simulink model "pattern_separation"  (R2019b)
settings: Solver=FixedStepAuto  StartTime=1  StopTime=simulationtime  FixedStep=stepsize  RelTol=1e-3
values from neighbouring files (symbols this model uses):
  a1 = 0.02    [simulation.m]
  a2 = 0.02    [simulation.m]
  b1 = 0.025    [simulation.m]
  b2 = 0.04    [simulation.m]
  c1 = -65    [simulation.m]
  C1 = normrnd(100,10,[1,nrofgranulecells])    [simulation.m]
  c2 = -65    [simulation.m]
  C2 = normrnd(100,10,[1,nrofinterneurons])    [simulation.m]
  d1 = 6    [simulation.m]
  d2 = 2    [simulation.m]
  inputset = inputsets{no_input}    [simulation.m]
  k1 = 0.25    [simulation.m]
  k2 = 0.25    [simulation.m]
  minimum_saturation_limit_1 = -80    [simulation.m]
  minimum_saturation_limit_2 = -100    [simulation.m]
  noumberofevents = 500    [simulation.m]
  Re = 230    [simulation.m]
  simulationtime = 2000    [simulation.m]
  stepsize = 1    [simulation.m]
  ve1 = -5    [simulation.m]
  ve2 = -80    [simulation.m]
  vr1 = -60    [simulation.m]
  vr2 = -65    [simulation.m]
  vt1 = -55    [simulation.m]
  vt2 = -48    [simulation.m]
undefined symbols (not defined in the file or in its folder): conductancemaxima1, conductancemaxima2, conductancemaxima3, decaytimes1, decaytimes2, decaytimes3, DiscIntNeverNeededParam, Nd, trace
(part 2 of 5)

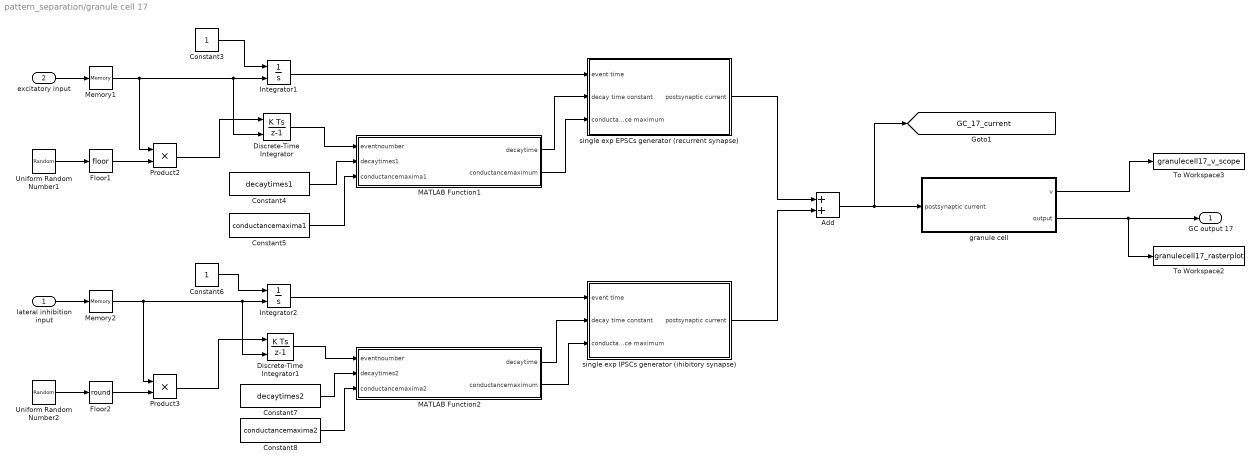
== system pattern_separation/granule cell 17 ==
  lateral inhibition input : Inport
  excitatory input : Inport  Port=2
  Add : Sum
  Constant3 : Constant  SampleTime=-1
  Constant4 : Constant  Value=decaytimes1  SampleTime=-1
  Constant5 : Constant  Value=conductancemaxima1  SampleTime=-1
  Constant6 : Constant  SampleTime=-1
  Constant7 : Constant  Value=decaytimes2  SampleTime=-1
  Constant8 : Constant  Value=conductancemaxima2  SampleTime=-1
  Discrete-Time Integrator : DiscreteIntegrator  gainval=1/stepsize  ExternalReset=sampled level  SampleTime=-1  ICPrevOutput=DiscIntNeverNeededParam  ICPrevScaledInput=DiscIntNeverNeededParam
  Discrete-Time Integrator1 : DiscreteIntegrator  gainval=1/stepsize  ExternalReset=sampled level  SampleTime=-1  ICPrevOutput=DiscIntNeverNeededParam  ICPrevScaledInput=DiscIntNeverNeededParam
  Floor1 : Rounding
  Floor2 : Rounding  Operator=round
  Integrator1 : Integrator  ExternalReset=level hold
  Integrator2 : Integrator  ExternalReset=level hold
  MATLAB Function1 : MATLAB Function  TreatAsAtomicUnit=on
  MATLAB Function2 : MATLAB Function  TreatAsAtomicUnit=on
  Memory1 : Memory  InheritSampleTime=on
  Memory2 : Memory  InheritSampleTime=on
  Product2 : Product
  Product3 : Product
  To Workspace2 : ToWorkspace  VariableName=granulecell17_rasterplot  SampleTime=-1
  To Workspace3 : ToWorkspace  VariableName=granulecell17_v_scope  SampleTime=-1
  Uniform Random Number1 : UniformRandomNumber  Minimum=1  Maximum=noumberofevents  Seed=33  SampleTime=stepsize
  Uniform Random Number2 : UniformRandomNumber  Minimum=1  Maximum=noumberofevents  Seed=34  SampleTime=stepsize
  granule cell : Subsystem
  single exp EPSCs generator (recurrent synapse) : Subsystem
  single exp IPSCs generator (ihibitory synapse) : Subsystem
  GC output 17 : Outport
  tag scope: GC_17_current=global
  wires:
  Discrete-Time Integrator/1 -> MATLAB Function1/1(eventnoumber)
  Memory1/1 -> Product2/1, Discrete-Time Integrator/2, Integrator1/2
  granule cell/2(output) -> GC output 17/1, To Workspace2/1
  MATLAB Function2/2(conductancemaximum) -> single exp IPSCs generator (ihibitory synapse)/3(conductance maximum)
  lateral inhibition input/1 -> Memory2/1
  Uniform Random Number1/1 -> Floor1/1
  Uniform Random Number2/1 -> Floor2/1
  excitatory input/1 -> Memory1/1
  single exp EPSCs generator (recurrent synapse)/1(postsynaptic current) -> Add/1
  Product3/1 -> Discrete-Time Integrator1/1
  Floor1/1 -> Product2/2
  Constant3/1 -> Integrator1/1
  single exp IPSCs generator (ihibitory synapse)/1(postsynaptic current) -> Add/2
  Product2/1 -> Discrete-Time Integrator/1
  granule cell/1(v) -> To Workspace3/1
  MATLAB Function1/1(decaytime) -> single exp EPSCs generator (recurrent synapse)/2(decay time constant)
  MATLAB Function2/1(decaytime) -> single exp IPSCs generator (ihibitory synapse)/2(decay time constant)
  Add/1 -> [GC_17_current], granule cell/1(postsynaptic current)
  Integrator1/1 -> single exp EPSCs generator (recurrent synapse)/1(event time)
  Constant5/1 -> MATLAB Function1/3(conductancemaxima1)
  Memory2/1 -> Product3/1, Discrete-Time Integrator1/2, Integrator2/2
  MATLAB Function1/2(conductancemaximum) -> single exp EPSCs generator (recurrent synapse)/3(conductance maximum)
  Constant6/1 -> Integrator2/1
  Constant4/1 -> MATLAB Function1/2(decaytimes1)
  Constant7/1 -> MATLAB Function2/2(decaytimes2)
  Constant8/1 -> MATLAB Function2/3(conductancemaxima2)
  Floor2/1 -> Product3/2
  Integrator2/1 -> single exp IPSCs generator (ihibitory synapse)/1(event time)
  Discrete-Time Integrator1/1 -> MATLAB Function2/1(eventnoumber)

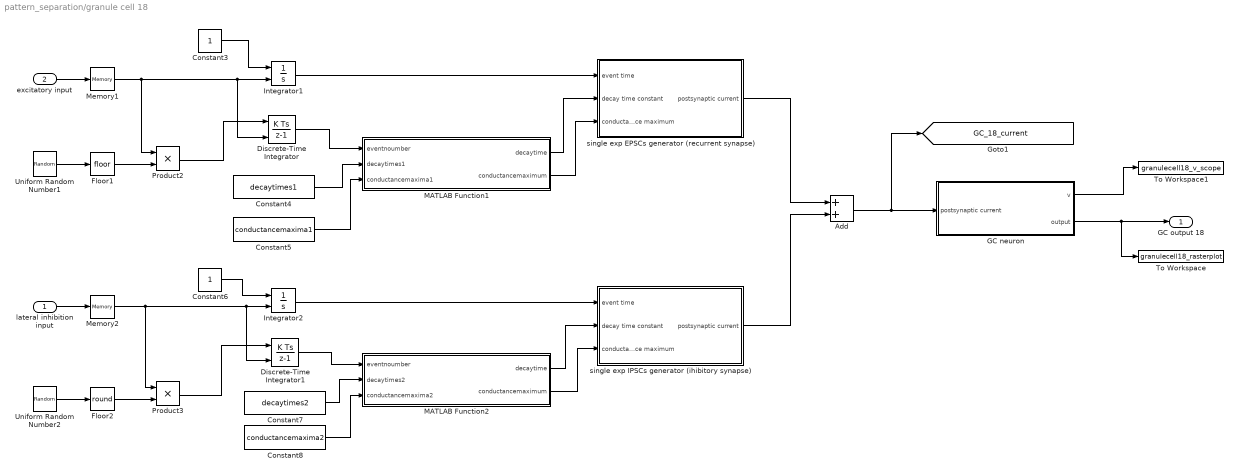
== system pattern_separation/granule cell 18 ==
  lateral inhibition input : Inport
  excitatory input : Inport  Port=2
  Add : Sum
  Constant3 : Constant  SampleTime=-1
  Constant4 : Constant  Value=decaytimes1  SampleTime=-1
  Constant5 : Constant  Value=conductancemaxima1  SampleTime=-1
  Constant6 : Constant  SampleTime=-1
  Constant7 : Constant  Value=decaytimes2  SampleTime=-1
  Constant8 : Constant  Value=conductancemaxima2  VectorParams1D=off  SampleTime=-1
  Discrete-Time Integrator : DiscreteIntegrator  gainval=1/stepsize  ExternalReset=sampled level  SampleTime=-1  ICPrevOutput=DiscIntNeverNeededParam  ICPrevScaledInput=DiscIntNeverNeededParam
  Discrete-Time Integrator1 : DiscreteIntegrator  gainval=1/stepsize  ExternalReset=sampled level  SampleTime=-1  ICPrevOutput=DiscIntNeverNeededParam  ICPrevScaledInput=DiscIntNeverNeededParam
  Floor1 : Rounding
  Floor2 : Rounding  Operator=round
  GC neuron : Subsystem
  Integrator1 : Integrator  ExternalReset=level hold
  Integrator2 : Integrator  ExternalReset=level hold
  MATLAB Function1 : MATLAB Function  TreatAsAtomicUnit=on
  MATLAB Function2 : MATLAB Function  TreatAsAtomicUnit=on
  Memory1 : Memory  InheritSampleTime=on
  Memory2 : Memory  InheritSampleTime=on
  Product2 : Product
  Product3 : Product
  To Workspace : ToWorkspace  VariableName=granulecell18_rasterplot  SampleTime=-1
  To Workspace1 : ToWorkspace  VariableName=granulecell18_v_scope  SampleTime=-1
  Uniform Random Number1 : UniformRandomNumber  Minimum=1  Maximum=noumberofevents  Seed=35  SampleTime=stepsize
  Uniform Random Number2 : UniformRandomNumber  Minimum=1  Maximum=noumberofevents  Seed=36  SampleTime=stepsize
  single exp EPSCs generator (recurrent synapse) : Subsystem
  single exp IPSCs generator (ihibitory synapse) : Subsystem
  GC output 18 : Outport
  tag scope: GC_18_current=global
  wires:
  GC neuron/1(v) -> To Workspace1/1
  GC neuron/2(output) -> To Workspace/1, GC output 18/1
  Constant7/1 -> MATLAB Function2/2(decaytimes2)
  Constant8/1 -> MATLAB Function2/3(conductancemaxima2)
  Discrete-Time Integrator1/1 -> MATLAB Function2/1(eventnoumber)
  Floor2/1 -> Product3/2
  Discrete-Time Integrator/1 -> MATLAB Function1/1(eventnoumber)
  MATLAB Function2/1(decaytime) -> single exp IPSCs generator (ihibitory synapse)/2(decay time constant)
  Product2/1 -> Discrete-Time Integrator/1
  Integrator2/1 -> single exp IPSCs generator (ihibitory synapse)/1(event time)
  Add/1 -> [GC_18_current], GC neuron/1(postsynaptic current)
  Memory2/1 -> Product3/1, Discrete-Time Integrator1/2, Integrator2/2
  single exp IPSCs generator (ihibitory synapse)/1(postsynaptic current) -> Add/2
  MATLAB Function1/1(decaytime) -> single exp EPSCs generator (recurrent synapse)/2(decay time constant)
  MATLAB Function1/2(conductancemaximum) -> single exp EPSCs generator (recurrent synapse)/3(conductance maximum)
  Constant6/1 -> Integrator2/1
  Constant4/1 -> MATLAB Function1/2(decaytimes1)
  Constant5/1 -> MATLAB Function1/3(conductancemaxima1)
  Integrator1/1 -> single exp EPSCs generator (recurrent synapse)/1(event time)
  Product3/1 -> Discrete-Time Integrator1/1
  single exp EPSCs generator (recurrent synapse)/1(postsynaptic current) -> Add/1
  lateral inhibition input/1 -> Memory2/1
  Floor1/1 -> Product2/2
  MATLAB Function2/2(conductancemaximum) -> single exp IPSCs generator (ihibitory synapse)/3(conductance maximum)
  Memory1/1 -> Product2/1, Discrete-Time Integrator/2, Integrator1/2
  Uniform Random Number1/1 -> Floor1/1
  Constant3/1 -> Integrator1/1
  Uniform Random Number2/1 -> Floor2/1
  excitatory input/1 -> Memory1/1

== system pattern_separation/granule cell 19 ==
  lateral inhibition input : Inport
  excitatory input : Inport  Port=2
  Add : Sum
  Constant3 : Constant  SampleTime=-1
  Constant4 : Constant  Value=decaytimes1  SampleTime=-1
  Constant5 : Constant  Value=conductancemaxima1  SampleTime=-1
  Constant6 : Constant  SampleTime=-1
  Constant7 : Constant  Value=decaytimes2  SampleTime=-1
  Constant8 : Constant  Value=conductancemaxima2  SampleTime=-1
  Discrete-Time Integrator : DiscreteIntegrator  gainval=1/stepsize  ExternalReset=sampled level  SampleTime=-1  ICPrevOutput=DiscIntNeverNeededParam  ICPrevScaledInput=DiscIntNeverNeededParam
  Discrete-Time Integrator1 : DiscreteIntegrator  gainval=1/stepsize  ExternalReset=sampled level  SampleTime=-1  ICPrevOutput=DiscIntNeverNeededParam  ICPrevScaledInput=DiscIntNeverNeededParam
  Floor1 : Rounding
  Floor2 : Rounding  Operator=round
  Integrator1 : Integrator  ExternalReset=level hold
  Integrator2 : Integrator  ExternalReset=level hold
  MATLAB Function1 : MATLAB Function  TreatAsAtomicUnit=on
  MATLAB Function2 : MATLAB Function  TreatAsAtomicUnit=on
  Memory1 : Memory  InheritSampleTime=on
  Memory2 : Memory  InheritSampleTime=on
  Product2 : Product
  Product3 : Product
  To Workspace2 : ToWorkspace  VariableName=granulecell19_rasterplot  SampleTime=-1
  To Workspace3 : ToWorkspace  VariableName=granulecell19_v_scope  SampleTime=-1
  Uniform Random Number1 : UniformRandomNumber  Minimum=1  Maximum=noumberofevents  Seed=37  SampleTime=stepsize
  Uniform Random Number2 : UniformRandomNumber  Minimum=1  Maximum=noumberofevents  Seed=38  SampleTime=stepsize
  granule cell : Subsystem
  single exp EPSCs generator (recurrent synapse) : Subsystem
  single exp IPSCs generator (ihibitory synapse) : Subsystem
  GC output 19 : Outport
  tag scope: GC_19_current=global
  wires:
  Discrete-Time Integrator/1 -> MATLAB Function1/1(eventnoumber)
  Memory1/1 -> Product2/1, Discrete-Time Integrator/2, Integrator1/2
  granule cell/2(output) -> GC output 19/1, To Workspace2/1
  MATLAB Function2/2(conductancemaximum) -> single exp IPSCs generator (ihibitory synapse)/3(conductance maximum)
  lateral inhibition input/1 -> Memory2/1
  Uniform Random Number1/1 -> Floor1/1
  Uniform Random Number2/1 -> Floor2/1
  excitatory input/1 -> Memory1/1
  single exp EPSCs generator (recurrent synapse)/1(postsynaptic current) -> Add/1
  Product3/1 -> Discrete-Time Integrator1/1
  Floor1/1 -> Product2/2
  Constant3/1 -> Integrator1/1
  single exp IPSCs generator (ihibitory synapse)/1(postsynaptic current) -> Add/2
  Product2/1 -> Discrete-Time Integrator/1
  granule cell/1(v) -> To Workspace3/1
  MATLAB Function1/1(decaytime) -> single exp EPSCs generator (recurrent synapse)/2(decay time constant)
  MATLAB Function2/1(decaytime) -> single exp IPSCs generator (ihibitory synapse)/2(decay time constant)
  Add/1 -> [GC_19_current], granule cell/1(postsynaptic current)
  Integrator1/1 -> single exp EPSCs generator (recurrent synapse)/1(event time)
  Constant5/1 -> MATLAB Function1/3(conductancemaxima1)
  Memory2/1 -> Product3/1, Discrete-Time Integrator1/2, Integrator2/2
  MATLAB Function1/2(conductancemaximum) -> single exp EPSCs generator (recurrent synapse)/3(conductance maximum)
  Constant6/1 -> Integrator2/1
  Constant4/1 -> MATLAB Function1/2(decaytimes1)
  Constant7/1 -> MATLAB Function2/2(decaytimes2)
  Constant8/1 -> MATLAB Function2/3(conductancemaxima2)
  Floor2/1 -> Product3/2
  Integrator2/1 -> single exp IPSCs generator (ihibitory synapse)/1(event time)
  Discrete-Time Integrator1/1 -> MATLAB Function2/1(eventnoumber)

== system pattern_separation/granule cell 2 ==
  lateral inhibition input : Inport
  excitatory input : Inport  Port=2
  Add : Sum
  Constant3 : Constant  SampleTime=-1
  Constant4 : Constant  Value=decaytimes1  SampleTime=-1
  Constant5 : Constant  Value=conductancemaxima1  SampleTime=-1
  Constant6 : Constant  SampleTime=-1
  Constant7 : Constant  Value=decaytimes2  SampleTime=-1
  Constant8 : Constant  Value=conductancemaxima2  VectorParams1D=off  SampleTime=-1
  Discrete-Time Integrator : DiscreteIntegrator  gainval=1/stepsize  ExternalReset=sampled level  SampleTime=-1  ICPrevOutput=DiscIntNeverNeededParam  ICPrevScaledInput=DiscIntNeverNeededParam
  Discrete-Time Integrator1 : DiscreteIntegrator  gainval=1/stepsize  ExternalReset=sampled level  SampleTime=-1  ICPrevOutput=DiscIntNeverNeededParam  ICPrevScaledInput=DiscIntNeverNeededParam
  Floor1 : Rounding
  Floor2 : Rounding  Operator=round
  GC neuron : Subsystem
  Integrator1 : Integrator  ExternalReset=level hold
  Integrator2 : Integrator  ExternalReset=level hold
  MATLAB Function1 : MATLAB Function  TreatAsAtomicUnit=on
  MATLAB Function2 : MATLAB Function  TreatAsAtomicUnit=on
  Memory1 : Memory  InheritSampleTime=on
  Memory2 : Memory  InheritSampleTime=on
  Product2 : Product
  Product3 : Product
  To Workspace : ToWorkspace  VariableName=granulecell2_rasterplot  SampleTime=-1
  To Workspace1 : ToWorkspace  VariableName=granulecell2_v_scope  SampleTime=-1
  Uniform Random Number1 : UniformRandomNumber  Minimum=1  Maximum=noumberofevents  Seed=3  SampleTime=stepsize
  Uniform Random Number2 : UniformRandomNumber  Minimum=1  Maximum=noumberofevents  Seed=4  SampleTime=stepsize
  single exp EPSCs generator (recurrent synapse) : Subsystem
  single exp IPSCs generator (ihibitory synapse) : Subsystem
  GC output 2 : Outport
  tag scope: GC_2_current=global
  wires:
  GC neuron/1(v) -> To Workspace1/1
  GC neuron/2(output) -> To Workspace/1, GC output 2/1
  Constant7/1 -> MATLAB Function2/2(decaytimes2)
  Constant8/1 -> MATLAB Function2/3(conductancemaxima2)
  Discrete-Time Integrator1/1 -> MATLAB Function2/1(eventnoumber)
  Floor2/1 -> Product3/2
  Discrete-Time Integrator/1 -> MATLAB Function1/1(eventnoumber)
  MATLAB Function2/1(decaytime) -> single exp IPSCs generator (ihibitory synapse)/2(decay time constant)
  Product2/1 -> Discrete-Time Integrator/1
  Integrator2/1 -> single exp IPSCs generator (ihibitory synapse)/1(event time)
  Add/1 -> [GC_2_current], GC neuron/1(postsynaptic current)
  Memory2/1 -> Product3/1, Discrete-Time Integrator1/2, Integrator2/2
  single exp IPSCs generator (ihibitory synapse)/1(postsynaptic current) -> Add/2
  MATLAB Function1/1(decaytime) -> single exp EPSCs generator (recurrent synapse)/2(decay time constant)
  MATLAB Function1/2(conductancemaximum) -> single exp EPSCs generator (recurrent synapse)/3(conductance maximum)
  Constant6/1 -> Integrator2/1
  Constant4/1 -> MATLAB Function1/2(decaytimes1)
  Constant5/1 -> MATLAB Function1/3(conductancemaxima1)
  Integrator1/1 -> single exp EPSCs generator (recurrent synapse)/1(event time)
  Product3/1 -> Discrete-Time Integrator1/1
  single exp EPSCs generator (recurrent synapse)/1(postsynaptic current) -> Add/1
  lateral inhibition input/1 -> Memory2/1
  Floor1/1 -> Product2/2
  MATLAB Function2/2(conductancemaximum) -> single exp IPSCs generator (ihibitory synapse)/3(conductance maximum)
  Memory1/1 -> Product2/1, Discrete-Time Integrator/2, Integrator1/2
  Uniform Random Number1/1 -> Floor1/1
  Constant3/1 -> Integrator1/1
  Uniform Random Number2/1 -> Floor2/1
  excitatory input/1 -> Memory1/1

== system pattern_separation/granule cell 20 ==
  lateral inhibition input : Inport
  excitatory input : Inport  Port=2
  Add : Sum
  Constant3 : Constant  SampleTime=-1
  Constant4 : Constant  Value=decaytimes1  SampleTime=-1
  Constant5 : Constant  Value=conductancemaxima1  SampleTime=-1
  Constant6 : Constant  SampleTime=-1
  Constant7 : Constant  Value=decaytimes2  SampleTime=-1
  Constant8 : Constant  Value=conductancemaxima2  VectorParams1D=off  SampleTime=-1
  Discrete-Time Integrator : DiscreteIntegrator  gainval=1/stepsize  ExternalReset=sampled level  SampleTime=-1  ICPrevOutput=DiscIntNeverNeededParam  ICPrevScaledInput=DiscIntNeverNeededParam
  Discrete-Time Integrator1 : DiscreteIntegrator  gainval=1/stepsize  ExternalReset=sampled level  SampleTime=-1  ICPrevOutput=DiscIntNeverNeededParam  ICPrevScaledInput=DiscIntNeverNeededParam
  Floor1 : Rounding
  Floor2 : Rounding  Operator=round
  GC neuron : Subsystem
  Integrator1 : Integrator  ExternalReset=level hold
  Integrator2 : Integrator  ExternalReset=level hold
  MATLAB Function1 : MATLAB Function  TreatAsAtomicUnit=on
  MATLAB Function2 : MATLAB Function  TreatAsAtomicUnit=on
  Memory1 : Memory  InheritSampleTime=on
  Memory2 : Memory  InheritSampleTime=on
  Product2 : Product
  Product3 : Product
  To Workspace : ToWorkspace  VariableName=granulecell20_rasterplot  SampleTime=-1
  To Workspace1 : ToWorkspace  VariableName=granulecell20_v_scope  SampleTime=-1
  Uniform Random Number1 : UniformRandomNumber  Minimum=1  Maximum=noumberofevents  Seed=39  SampleTime=stepsize
  Uniform Random Number2 : UniformRandomNumber  Minimum=1  Maximum=noumberofevents  Seed=40  SampleTime=stepsize
  single exp EPSCs generator (recurrent synapse) : Subsystem
  single exp IPSCs generator (ihibitory synapse) : Subsystem
  GC output 20 : Outport
  tag scope: GC_20_current=global
  wires:
  GC neuron/1(v) -> To Workspace1/1
  GC neuron/2(output) -> To Workspace/1, GC output 20/1
  Constant7/1 -> MATLAB Function2/2(decaytimes2)
  Constant8/1 -> MATLAB Function2/3(conductancemaxima2)
  Discrete-Time Integrator1/1 -> MATLAB Function2/1(eventnoumber)
  Floor2/1 -> Product3/2
  Discrete-Time Integrator/1 -> MATLAB Function1/1(eventnoumber)
  MATLAB Function2/1(decaytime) -> single exp IPSCs generator (ihibitory synapse)/2(decay time constant)
  Product2/1 -> Discrete-Time Integrator/1
  Integrator2/1 -> single exp IPSCs generator (ihibitory synapse)/1(event time)
  Add/1 -> [GC_20_current], GC neuron/1(postsynaptic current)
  Memory2/1 -> Product3/1, Discrete-Time Integrator1/2, Integrator2/2
  single exp IPSCs generator (ihibitory synapse)/1(postsynaptic current) -> Add/2
  MATLAB Function1/1(decaytime) -> single exp EPSCs generator (recurrent synapse)/2(decay time constant)
  MATLAB Function1/2(conductancemaximum) -> single exp EPSCs generator (recurrent synapse)/3(conductance maximum)
  Constant6/1 -> Integrator2/1
  Constant4/1 -> MATLAB Function1/2(decaytimes1)
  Constant5/1 -> MATLAB Function1/3(conductancemaxima1)
  Integrator1/1 -> single exp EPSCs generator (recurrent synapse)/1(event time)
  Product3/1 -> Discrete-Time Integrator1/1
  single exp EPSCs generator (recurrent synapse)/1(postsynaptic current) -> Add/1
  lateral inhibition input/1 -> Memory2/1
  Floor1/1 -> Product2/2
  MATLAB Function2/2(conductancemaximum) -> single exp IPSCs generator (ihibitory synapse)/3(conductance maximum)
  Memory1/1 -> Product2/1, Discrete-Time Integrator/2, Integrator1/2
  Uniform Random Number1/1 -> Floor1/1
  Constant3/1 -> Integrator1/1
  Uniform Random Number2/1 -> Floor2/1
  excitatory input/1 -> Memory1/1

== system pattern_separation/granule cell 3 ==
  lateral inhibition input : Inport
  excitatory input : Inport  Port=2
  Add : Sum
  Constant3 : Constant  SampleTime=-1
  Constant4 : Constant  Value=decaytimes1  SampleTime=-1
  Constant5 : Constant  Value=conductancemaxima1  SampleTime=-1
  Constant6 : Constant  SampleTime=-1
  Constant7 : Constant  Value=decaytimes2  SampleTime=-1
  Constant8 : Constant  Value=conductancemaxima2  VectorParams1D=off  SampleTime=-1
  Discrete-Time Integrator : DiscreteIntegrator  gainval=1/stepsize  ExternalReset=sampled level  SampleTime=-1  ICPrevOutput=DiscIntNeverNeededParam  ICPrevScaledInput=DiscIntNeverNeededParam
  Discrete-Time Integrator1 : DiscreteIntegrator  gainval=1/stepsize  ExternalReset=sampled level  SampleTime=-1  ICPrevOutput=DiscIntNeverNeededParam  ICPrevScaledInput=DiscIntNeverNeededParam
  Floor1 : Rounding
  Floor2 : Rounding  Operator=round
  GC neuron : Subsystem
  Integrator1 : Integrator  ExternalReset=level hold
  Integrator2 : Integrator  ExternalReset=level hold
  MATLAB Function1 : MATLAB Function  TreatAsAtomicUnit=on
  MATLAB Function2 : MATLAB Function  TreatAsAtomicUnit=on
  Memory1 : Memory  InheritSampleTime=on
  Memory2 : Memory  InheritSampleTime=on
  Product2 : Product
  Product3 : Product
  To Workspace : ToWorkspace  VariableName=granulecell3_rasterplot  SampleTime=-1
  To Workspace1 : ToWorkspace  VariableName=granulecell3_v_scope  SampleTime=-1
  Uniform Random Number1 : UniformRandomNumber  Minimum=1  Maximum=noumberofevents  Seed=5  SampleTime=stepsize
  Uniform Random Number2 : UniformRandomNumber  Minimum=1  Maximum=noumberofevents  Seed=6  SampleTime=stepsize
  single exp EPSCs generator (recurrent synapse) : Subsystem
  single exp IPSCs generator (ihibitory synapse) : Subsystem
  GC output 3 : Outport
  tag scope: GC_3_current=global
  wires:
  GC neuron/1(v) -> To Workspace1/1
  GC neuron/2(output) -> To Workspace/1, GC output 3/1
  Constant7/1 -> MATLAB Function2/2(decaytimes2)
  Constant8/1 -> MATLAB Function2/3(conductancemaxima2)
  Discrete-Time Integrator1/1 -> MATLAB Function2/1(eventnoumber)
  Floor2/1 -> Product3/2
  Discrete-Time Integrator/1 -> MATLAB Function1/1(eventnoumber)
  MATLAB Function2/1(decaytime) -> single exp IPSCs generator (ihibitory synapse)/2(decay time constant)
  Product2/1 -> Discrete-Time Integrator/1
  Integrator2/1 -> single exp IPSCs generator (ihibitory synapse)/1(event time)
  Add/1 -> [GC_3_current], GC neuron/1(postsynaptic current)
  Memory2/1 -> Product3/1, Discrete-Time Integrator1/2, Integrator2/2
  single exp IPSCs generator (ihibitory synapse)/1(postsynaptic current) -> Add/2
  MATLAB Function1/1(decaytime) -> single exp EPSCs generator (recurrent synapse)/2(decay time constant)
  MATLAB Function1/2(conductancemaximum) -> single exp EPSCs generator (recurrent synapse)/3(conductance maximum)
  Constant6/1 -> Integrator2/1
  Constant4/1 -> MATLAB Function1/2(decaytimes1)
  Constant5/1 -> MATLAB Function1/3(conductancemaxima1)
  Integrator1/1 -> single exp EPSCs generator (recurrent synapse)/1(event time)
  Product3/1 -> Discrete-Time Integrator1/1
  single exp EPSCs generator (recurrent synapse)/1(postsynaptic current) -> Add/1
  lateral inhibition input/1 -> Memory2/1
  Floor1/1 -> Product2/2
  MATLAB Function2/2(conductancemaximum) -> single exp IPSCs generator (ihibitory synapse)/3(conductance maximum)
  Memory1/1 -> Product2/1, Discrete-Time Integrator/2, Integrator1/2
  Uniform Random Number1/1 -> Floor1/1
  Constant3/1 -> Integrator1/1
  Uniform Random Number2/1 -> Floor2/1
  excitatory input/1 -> Memory1/1

== system pattern_separation/granule cell 4 ==
  lateral inhibition input : Inport
  excitatory input : Inport  Port=2
  Add : Sum
  Constant3 : Constant  SampleTime=-1
  Constant4 : Constant  Value=decaytimes1  SampleTime=-1
  Constant5 : Constant  Value=conductancemaxima1  SampleTime=-1
  Constant6 : Constant  SampleTime=-1
  Constant7 : Constant  Value=decaytimes2  SampleTime=-1
  Constant8 : Constant  Value=conductancemaxima2  VectorParams1D=off  SampleTime=-1
  Discrete-Time Integrator : DiscreteIntegrator  gainval=1/stepsize  ExternalReset=sampled level  SampleTime=-1  ICPrevOutput=DiscIntNeverNeededParam  ICPrevScaledInput=DiscIntNeverNeededParam
  Discrete-Time Integrator1 : DiscreteIntegrator  gainval=1/stepsize  ExternalReset=sampled level  SampleTime=-1  ICPrevOutput=DiscIntNeverNeededParam  ICPrevScaledInput=DiscIntNeverNeededParam
  Floor1 : Rounding
  Floor2 : Rounding  Operator=round
  GC neuron : Subsystem
  Integrator1 : Integrator  ExternalReset=level hold
  Integrator2 : Integrator  ExternalReset=level hold
  MATLAB Function1 : MATLAB Function  TreatAsAtomicUnit=on
  MATLAB Function2 : MATLAB Function  TreatAsAtomicUnit=on
  Memory1 : Memory  InheritSampleTime=on
  Memory2 : Memory  InheritSampleTime=on
  Product2 : Product
  Product3 : Product
  To Workspace : ToWorkspace  VariableName=granulecell4_rasterplot  SampleTime=-1
  To Workspace1 : ToWorkspace  VariableName=granulecell4_v_scope  SampleTime=-1
  Uniform Random Number1 : UniformRandomNumber  Minimum=1  Maximum=noumberofevents  Seed=7  SampleTime=stepsize
  Uniform Random Number2 : UniformRandomNumber  Minimum=1  Maximum=noumberofevents  Seed=8  SampleTime=stepsize
  single exp EPSCs generator (recurrent synapse) : Subsystem
  single exp IPSCs generator (ihibitory synapse) : Subsystem
  GC output 4 : Outport
  tag scope: GC_4_current=global
  wires:
  GC neuron/1(v) -> To Workspace1/1
  GC neuron/2(output) -> To Workspace/1, GC output 4/1
  Constant7/1 -> MATLAB Function2/2(decaytimes2)
  Constant8/1 -> MATLAB Function2/3(conductancemaxima2)
  Discrete-Time Integrator1/1 -> MATLAB Function2/1(eventnoumber)
  Floor2/1 -> Product3/2
  Discrete-Time Integrator/1 -> MATLAB Function1/1(eventnoumber)
  MATLAB Function2/1(decaytime) -> single exp IPSCs generator (ihibitory synapse)/2(decay time constant)
  Product2/1 -> Discrete-Time Integrator/1
  Integrator2/1 -> single exp IPSCs generator (ihibitory synapse)/1(event time)
  Add/1 -> [GC_4_current], GC neuron/1(postsynaptic current)
  Memory2/1 -> Product3/1, Discrete-Time Integrator1/2, Integrator2/2
  single exp IPSCs generator (ihibitory synapse)/1(postsynaptic current) -> Add/2
  MATLAB Function1/1(decaytime) -> single exp EPSCs generator (recurrent synapse)/2(decay time constant)
  MATLAB Function1/2(conductancemaximum) -> single exp EPSCs generator (recurrent synapse)/3(conductance maximum)
  Constant6/1 -> Integrator2/1
  Constant4/1 -> MATLAB Function1/2(decaytimes1)
  Constant5/1 -> MATLAB Function1/3(conductancemaxima1)
  Integrator1/1 -> single exp EPSCs generator (recurrent synapse)/1(event time)
  Product3/1 -> Discrete-Time Integrator1/1
  single exp EPSCs generator (recurrent synapse)/1(postsynaptic current) -> Add/1
  lateral inhibition input/1 -> Memory2/1
  Floor1/1 -> Product2/2
  MATLAB Function2/2(conductancemaximum) -> single exp IPSCs generator (ihibitory synapse)/3(conductance maximum)
  Memory1/1 -> Product2/1, Discrete-Time Integrator/2, Integrator1/2
  Uniform Random Number1/1 -> Floor1/1
  Constant3/1 -> Integrator1/1
  Uniform Random Number2/1 -> Floor2/1
  excitatory input/1 -> Memory1/1

== system pattern_separation/granule cell 5 ==
  lateral inhibition input : Inport
  excitatory input : Inport  Port=2
  Add : Sum
  Constant3 : Constant  SampleTime=-1
  Constant4 : Constant  Value=decaytimes1  SampleTime=-1
  Constant5 : Constant  Value=conductancemaxima1  SampleTime=-1
  Constant6 : Constant  SampleTime=-1
  Constant7 : Constant  Value=decaytimes2  SampleTime=-1
  Constant8 : Constant  Value=conductancemaxima2  SampleTime=-1
  Discrete-Time Integrator : DiscreteIntegrator  gainval=1/stepsize  ExternalReset=sampled level  SampleTime=-1  ICPrevOutput=DiscIntNeverNeededParam  ICPrevScaledInput=DiscIntNeverNeededParam
  Discrete-Time Integrator1 : DiscreteIntegrator  gainval=1/stepsize  ExternalReset=sampled level  SampleTime=-1  ICPrevOutput=DiscIntNeverNeededParam  ICPrevScaledInput=DiscIntNeverNeededParam
  Floor1 : Rounding
  Floor2 : Rounding  Operator=round
  Integrator1 : Integrator  ExternalReset=level hold
  Integrator2 : Integrator  ExternalReset=level hold
  MATLAB Function1 : MATLAB Function  TreatAsAtomicUnit=on
  MATLAB Function2 : MATLAB Function  TreatAsAtomicUnit=on
  Memory1 : Memory  InheritSampleTime=on
  Memory2 : Memory  InheritSampleTime=on
  Product2 : Product
  Product3 : Product
  To Workspace2 : ToWorkspace  VariableName=granulecell5_rasterplot  SampleTime=-1
  To Workspace3 : ToWorkspace  VariableName=granulecell5_v_scope  SampleTime=-1
  Uniform Random Number1 : UniformRandomNumber  Minimum=1  Maximum=noumberofevents  Seed=9  SampleTime=stepsize
  Uniform Random Number2 : UniformRandomNumber  Minimum=1  Maximum=noumberofevents  Seed=10  SampleTime=stepsize
  granule cell : Subsystem
  single exp EPSCs generator (recurrent synapse) : Subsystem
  single exp IPSCs generator (ihibitory synapse) : Subsystem
  GC output 5 : Outport
  tag scope: GC_5_current=global
  wires:
  Discrete-Time Integrator/1 -> MATLAB Function1/1(eventnoumber)
  Memory1/1 -> Product2/1, Discrete-Time Integrator/2, Integrator1/2
  granule cell/2(output) -> GC output 5/1, To Workspace2/1
  MATLAB Function2/2(conductancemaximum) -> single exp IPSCs generator (ihibitory synapse)/3(conductance maximum)
  lateral inhibition input/1 -> Memory2/1
  Uniform Random Number1/1 -> Floor1/1
  Uniform Random Number2/1 -> Floor2/1
  excitatory input/1 -> Memory1/1
  single exp EPSCs generator (recurrent synapse)/1(postsynaptic current) -> Add/1
  Product3/1 -> Discrete-Time Integrator1/1
  Floor1/1 -> Product2/2
  Constant3/1 -> Integrator1/1
  single exp IPSCs generator (ihibitory synapse)/1(postsynaptic current) -> Add/2
  Product2/1 -> Discrete-Time Integrator/1
  granule cell/1(v) -> To Workspace3/1
  MATLAB Function1/1(decaytime) -> single exp EPSCs generator (recurrent synapse)/2(decay time constant)
  MATLAB Function2/1(decaytime) -> single exp IPSCs generator (ihibitory synapse)/2(decay time constant)
  Add/1 -> [GC_5_current], granule cell/1(postsynaptic current)
  Integrator1/1 -> single exp EPSCs generator (recurrent synapse)/1(event time)
  Constant5/1 -> MATLAB Function1/3(conductancemaxima1)
  Memory2/1 -> Product3/1, Discrete-Time Integrator1/2, Integrator2/2
  MATLAB Function1/2(conductancemaximum) -> single exp EPSCs generator (recurrent synapse)/3(conductance maximum)
  Constant6/1 -> Integrator2/1
  Constant4/1 -> MATLAB Function1/2(decaytimes1)
  Constant7/1 -> MATLAB Function2/2(decaytimes2)
  Constant8/1 -> MATLAB Function2/3(conductancemaxima2)
  Floor2/1 -> Product3/2
  Integrator2/1 -> single exp IPSCs generator (ihibitory synapse)/1(event time)
  Discrete-Time Integrator1/1 -> MATLAB Function2/1(eventnoumber)

== system pattern_separation/granule cell 6 ==
  lateral inhibition input : Inport
  excitatory input : Inport  Port=2
  Add : Sum
  Constant3 : Constant  SampleTime=-1
  Constant4 : Constant  Value=decaytimes1  SampleTime=-1
  Constant5 : Constant  Value=conductancemaxima1  SampleTime=-1
  Constant6 : Constant  SampleTime=-1
  Constant7 : Constant  Value=decaytimes2  SampleTime=-1
  Constant8 : Constant  Value=conductancemaxima2  VectorParams1D=off  SampleTime=-1
  Discrete-Time Integrator : DiscreteIntegrator  gainval=1/stepsize  ExternalReset=sampled level  SampleTime=-1  ICPrevOutput=DiscIntNeverNeededParam  ICPrevScaledInput=DiscIntNeverNeededParam
  Discrete-Time Integrator1 : DiscreteIntegrator  gainval=1/stepsize  ExternalReset=sampled level  SampleTime=-1  ICPrevOutput=DiscIntNeverNeededParam  ICPrevScaledInput=DiscIntNeverNeededParam
  Floor1 : Rounding
  Floor2 : Rounding  Operator=round
  GC neuron : Subsystem
  Integrator1 : Integrator  ExternalReset=level hold
  Integrator2 : Integrator  ExternalReset=level hold
  MATLAB Function1 : MATLAB Function  TreatAsAtomicUnit=on
  MATLAB Function2 : MATLAB Function  TreatAsAtomicUnit=on
  Memory1 : Memory  InheritSampleTime=on
  Memory2 : Memory  InheritSampleTime=on
  Product2 : Product
  Product3 : Product
  To Workspace : ToWorkspace  VariableName=granulecell6_rasterplot  SampleTime=-1
  To Workspace1 : ToWorkspace  VariableName=granulecell6_v_scope  SampleTime=-1
  Uniform Random Number1 : UniformRandomNumber  Minimum=1  Maximum=noumberofevents  Seed=11  SampleTime=stepsize
  Uniform Random Number2 : UniformRandomNumber  Minimum=1  Maximum=noumberofevents  Seed=12  SampleTime=stepsize
  single exp EPSCs generator (recurrent synapse) : Subsystem
  single exp IPSCs generator (ihibitory synapse) : Subsystem
  GC output 6 : Outport
  tag scope: GC_6_current=global
  wires:
  GC neuron/1(v) -> To Workspace1/1
  GC neuron/2(output) -> To Workspace/1, GC output 6/1
  Constant7/1 -> MATLAB Function2/2(decaytimes2)
  Constant8/1 -> MATLAB Function2/3(conductancemaxima2)
  Discrete-Time Integrator1/1 -> MATLAB Function2/1(eventnoumber)
  Floor2/1 -> Product3/2
  Discrete-Time Integrator/1 -> MATLAB Function1/1(eventnoumber)
  MATLAB Function2/1(decaytime) -> single exp IPSCs generator (ihibitory synapse)/2(decay time constant)
  Product2/1 -> Discrete-Time Integrator/1
  Integrator2/1 -> single exp IPSCs generator (ihibitory synapse)/1(event time)
  Add/1 -> [GC_6_current], GC neuron/1(postsynaptic current)
  Memory2/1 -> Product3/1, Discrete-Time Integrator1/2, Integrator2/2
  single exp IPSCs generator (ihibitory synapse)/1(postsynaptic current) -> Add/2
  MATLAB Function1/1(decaytime) -> single exp EPSCs generator (recurrent synapse)/2(decay time constant)
  MATLAB Function1/2(conductancemaximum) -> single exp EPSCs generator (recurrent synapse)/3(conductance maximum)
  Constant6/1 -> Integrator2/1
  Constant4/1 -> MATLAB Function1/2(decaytimes1)
  Constant5/1 -> MATLAB Function1/3(conductancemaxima1)
  Integrator1/1 -> single exp EPSCs generator (recurrent synapse)/1(event time)
  Product3/1 -> Discrete-Time Integrator1/1
  single exp EPSCs generator (recurrent synapse)/1(postsynaptic current) -> Add/1
  lateral inhibition input/1 -> Memory2/1
  Floor1/1 -> Product2/2
  MATLAB Function2/2(conductancemaximum) -> single exp IPSCs generator (ihibitory synapse)/3(conductance maximum)
  Memory1/1 -> Product2/1, Discrete-Time Integrator/2, Integrator1/2
  Uniform Random Number1/1 -> Floor1/1
  Constant3/1 -> Integrator1/1
  Uniform Random Number2/1 -> Floor2/1
  excitatory input/1 -> Memory1/1

== system pattern_separation/granule cell 7 ==
  lateral inhibition input : Inport
  excitatory input : Inport  Port=2
  Add : Sum
  Constant3 : Constant  SampleTime=-1
  Constant4 : Constant  Value=decaytimes1  SampleTime=-1
  Constant5 : Constant  Value=conductancemaxima1  SampleTime=-1
  Constant6 : Constant  SampleTime=-1
  Constant7 : Constant  Value=decaytimes2  SampleTime=-1
  Constant8 : Constant  Value=conductancemaxima2  SampleTime=-1
  Discrete-Time Integrator : DiscreteIntegrator  gainval=1/stepsize  ExternalReset=sampled level  SampleTime=-1  ICPrevOutput=DiscIntNeverNeededParam  ICPrevScaledInput=DiscIntNeverNeededParam
  Discrete-Time Integrator1 : DiscreteIntegrator  gainval=1/stepsize  ExternalReset=sampled level  SampleTime=-1  ICPrevOutput=DiscIntNeverNeededParam  ICPrevScaledInput=DiscIntNeverNeededParam
  Floor1 : Rounding
  Floor2 : Rounding  Operator=round
  Integrator1 : Integrator  ExternalReset=level hold
  Integrator2 : Integrator  ExternalReset=level hold
  MATLAB Function1 : MATLAB Function  TreatAsAtomicUnit=on
  MATLAB Function2 : MATLAB Function  TreatAsAtomicUnit=on
  Memory1 : Memory  InheritSampleTime=on
  Memory2 : Memory  InheritSampleTime=on
  Product2 : Product
  Product3 : Product
  To Workspace2 : ToWorkspace  VariableName=granulecell7_rasterplot  SampleTime=-1
  To Workspace3 : ToWorkspace  VariableName=granulecell7_v_scope  SampleTime=-1
  Uniform Random Number1 : UniformRandomNumber  Minimum=1  Maximum=noumberofevents  Seed=13  SampleTime=stepsize
  Uniform Random Number2 : UniformRandomNumber  Minimum=1  Maximum=noumberofevents  Seed=14  SampleTime=stepsize
  granule cell : Subsystem
  single exp EPSCs generator (recurrent synapse) : Subsystem
  single exp IPSCs generator (ihibitory synapse) : Subsystem
  GC output 7 : Outport
  tag scope: GC_7_current=global
  wires:
  Discrete-Time Integrator/1 -> MATLAB Function1/1(eventnoumber)
  Memory1/1 -> Product2/1, Discrete-Time Integrator/2, Integrator1/2
  granule cell/2(output) -> GC output 7/1, To Workspace2/1
  MATLAB Function2/2(conductancemaximum) -> single exp IPSCs generator (ihibitory synapse)/3(conductance maximum)
  lateral inhibition input/1 -> Memory2/1
  Uniform Random Number1/1 -> Floor1/1
  Uniform Random Number2/1 -> Floor2/1
  excitatory input/1 -> Memory1/1
  single exp EPSCs generator (recurrent synapse)/1(postsynaptic current) -> Add/1
  Product3/1 -> Discrete-Time Integrator1/1
  Floor1/1 -> Product2/2
  Constant3/1 -> Integrator1/1
  single exp IPSCs generator (ihibitory synapse)/1(postsynaptic current) -> Add/2
  Product2/1 -> Discrete-Time Integrator/1
  granule cell/1(v) -> To Workspace3/1
  MATLAB Function1/1(decaytime) -> single exp EPSCs generator (recurrent synapse)/2(decay time constant)
  MATLAB Function2/1(decaytime) -> single exp IPSCs generator (ihibitory synapse)/2(decay time constant)
  Add/1 -> [GC_7_current], granule cell/1(postsynaptic current)
  Integrator1/1 -> single exp EPSCs generator (recurrent synapse)/1(event time)
  Constant5/1 -> MATLAB Function1/3(conductancemaxima1)
  Memory2/1 -> Product3/1, Discrete-Time Integrator1/2, Integrator2/2
  MATLAB Function1/2(conductancemaximum) -> single exp EPSCs generator (recurrent synapse)/3(conductance maximum)
  Constant6/1 -> Integrator2/1
  Constant4/1 -> MATLAB Function1/2(decaytimes1)
  Constant7/1 -> MATLAB Function2/2(decaytimes2)
  Constant8/1 -> MATLAB Function2/3(conductancemaxima2)
  Floor2/1 -> Product3/2
  Integrator2/1 -> single exp IPSCs generator (ihibitory synapse)/1(event time)
  Discrete-Time Integrator1/1 -> MATLAB Function2/1(eventnoumber)

== system pattern_separation/granule cell 8 ==
  lateral inhibition input : Inport
  excitatory input : Inport  Port=2
  Add : Sum
  Constant3 : Constant  SampleTime=-1
  Constant4 : Constant  Value=decaytimes1  SampleTime=-1
  Constant5 : Constant  Value=conductancemaxima1  SampleTime=-1
  Constant6 : Constant  SampleTime=-1
  Constant7 : Constant  Value=decaytimes2  SampleTime=-1
  Constant8 : Constant  Value=conductancemaxima2  VectorParams1D=off  SampleTime=-1
  Discrete-Time Integrator : DiscreteIntegrator  gainval=1/stepsize  ExternalReset=sampled level  SampleTime=-1  ICPrevOutput=DiscIntNeverNeededParam  ICPrevScaledInput=DiscIntNeverNeededParam
  Discrete-Time Integrator1 : DiscreteIntegrator  gainval=1/stepsize  ExternalReset=sampled level  SampleTime=-1  ICPrevOutput=DiscIntNeverNeededParam  ICPrevScaledInput=DiscIntNeverNeededParam
  Floor1 : Rounding
  Floor2 : Rounding  Operator=round
  GC neuron : Subsystem
  Integrator1 : Integrator  ExternalReset=level hold
  Integrator2 : Integrator  ExternalReset=level hold
  MATLAB Function1 : MATLAB Function  TreatAsAtomicUnit=on
  MATLAB Function2 : MATLAB Function  TreatAsAtomicUnit=on
  Memory1 : Memory  InheritSampleTime=on
  Memory2 : Memory  InheritSampleTime=on
  Product2 : Product
  Product3 : Product
  To Workspace : ToWorkspace  VariableName=granulecell8_rasterplot  SampleTime=-1
  To Workspace1 : ToWorkspace  VariableName=granulecell8_v_scope  SampleTime=-1
  Uniform Random Number1 : UniformRandomNumber  Minimum=1  Maximum=noumberofevents  Seed=15  SampleTime=stepsize
  Uniform Random Number2 : UniformRandomNumber  Minimum=1  Maximum=noumberofevents  Seed=16  SampleTime=stepsize
  single exp EPSCs generator (recurrent synapse) : Subsystem
  single exp IPSCs generator (ihibitory synapse) : Subsystem
  GC output 8 : Outport
  tag scope: GC_8_current=global
  wires:
  GC neuron/1(v) -> To Workspace1/1
  GC neuron/2(output) -> To Workspace/1, GC output 8/1
  Constant7/1 -> MATLAB Function2/2(decaytimes2)
  Constant8/1 -> MATLAB Function2/3(conductancemaxima2)
  Discrete-Time Integrator1/1 -> MATLAB Function2/1(eventnoumber)
  Floor2/1 -> Product3/2
  Discrete-Time Integrator/1 -> MATLAB Function1/1(eventnoumber)
  MATLAB Function2/1(decaytime) -> single exp IPSCs generator (ihibitory synapse)/2(decay time constant)
  Product2/1 -> Discrete-Time Integrator/1
  Integrator2/1 -> single exp IPSCs generator (ihibitory synapse)/1(event time)
  Add/1 -> [GC_8_current], GC neuron/1(postsynaptic current)
  Memory2/1 -> Product3/1, Discrete-Time Integrator1/2, Integrator2/2
  single exp IPSCs generator (ihibitory synapse)/1(postsynaptic current) -> Add/2
  MATLAB Function1/1(decaytime) -> single exp EPSCs generator (recurrent synapse)/2(decay time constant)
  MATLAB Function1/2(conductancemaximum) -> single exp EPSCs generator (recurrent synapse)/3(conductance maximum)
  Constant6/1 -> Integrator2/1
  Constant4/1 -> MATLAB Function1/2(decaytimes1)
  Constant5/1 -> MATLAB Function1/3(conductancemaxima1)
  Integrator1/1 -> single exp EPSCs generator (recurrent synapse)/1(event time)
  Product3/1 -> Discrete-Time Integrator1/1
  single exp EPSCs generator (recurrent synapse)/1(postsynaptic current) -> Add/1
  lateral inhibition input/1 -> Memory2/1
  Floor1/1 -> Product2/2
  MATLAB Function2/2(conductancemaximum) -> single exp IPSCs generator (ihibitory synapse)/3(conductance maximum)
  Memory1/1 -> Product2/1, Discrete-Time Integrator/2, Integrator1/2
  Uniform Random Number1/1 -> Floor1/1
  Constant3/1 -> Integrator1/1
  Uniform Random Number2/1 -> Floor2/1
  excitatory input/1 -> Memory1/1

== system pattern_separation/granule cell 9 ==
  lateral inhibition input : Inport
  excitatory input : Inport  Port=2
  Add : Sum
  Constant3 : Constant  SampleTime=-1
  Constant4 : Constant  Value=decaytimes1  SampleTime=-1
  Constant5 : Constant  Value=conductancemaxima1  SampleTime=-1
  Constant6 : Constant  SampleTime=-1
  Constant7 : Constant  Value=decaytimes2  SampleTime=-1
  Constant8 : Constant  Value=conductancemaxima2  SampleTime=-1
  Discrete-Time Integrator : DiscreteIntegrator  gainval=1/stepsize  ExternalReset=sampled level  SampleTime=-1  ICPrevOutput=DiscIntNeverNeededParam  ICPrevScaledInput=DiscIntNeverNeededParam
  Discrete-Time Integrator1 : DiscreteIntegrator  gainval=1/stepsize  ExternalReset=sampled level  SampleTime=-1  ICPrevOutput=DiscIntNeverNeededParam  ICPrevScaledInput=DiscIntNeverNeededParam
  Floor1 : Rounding
  Floor2 : Rounding  Operator=round
  Integrator1 : Integrator  ExternalReset=level hold
  Integrator2 : Integrator  ExternalReset=level hold
  MATLAB Function1 : MATLAB Function  TreatAsAtomicUnit=on
  MATLAB Function2 : MATLAB Function  TreatAsAtomicUnit=on
  Memory1 : Memory  InheritSampleTime=on
  Memory2 : Memory  InheritSampleTime=on
  Product2 : Product
  Product3 : Product
  To Workspace2 : ToWorkspace  VariableName=granulecell9_rasterplot  SampleTime=-1
  To Workspace3 : ToWorkspace  VariableName=granulecell9_v_scope  SampleTime=-1
  Uniform Random Number1 : UniformRandomNumber  Minimum=1  Maximum=noumberofevents  Seed=17  SampleTime=stepsize
  Uniform Random Number2 : UniformRandomNumber  Minimum=1  Maximum=noumberofevents  Seed=18  SampleTime=stepsize
  granule cell : Subsystem
  single exp EPSCs generator (recurrent synapse) : Subsystem
  single exp IPSCs generator (ihibitory synapse) : Subsystem
  GC output 9 : Outport
  tag scope: GC_9_current=global
  wires:
  Discrete-Time Integrator/1 -> MATLAB Function1/1(eventnoumber)
  Memory1/1 -> Product2/1, Discrete-Time Integrator/2, Integrator1/2
  granule cell/2(output) -> GC output 9/1, To Workspace2/1
  MATLAB Function2/2(conductancemaximum) -> single exp IPSCs generator (ihibitory synapse)/3(conductance maximum)
  lateral inhibition input/1 -> Memory2/1
  Uniform Random Number1/1 -> Floor1/1
  Uniform Random Number2/1 -> Floor2/1
  excitatory input/1 -> Memory1/1
  single exp EPSCs generator (recurrent synapse)/1(postsynaptic current) -> Add/1
  Product3/1 -> Discrete-Time Integrator1/1
  Floor1/1 -> Product2/2
  Constant3/1 -> Integrator1/1
  single exp IPSCs generator (ihibitory synapse)/1(postsynaptic current) -> Add/2
  Product2/1 -> Discrete-Time Integrator/1
  granule cell/1(v) -> To Workspace3/1
  MATLAB Function1/1(decaytime) -> single exp EPSCs generator (recurrent synapse)/2(decay time constant)
  MATLAB Function2/1(decaytime) -> single exp IPSCs generator (ihibitory synapse)/2(decay time constant)
  Add/1 -> [GC_9_current], granule cell/1(postsynaptic current)
  Integrator1/1 -> single exp EPSCs generator (recurrent synapse)/1(event time)
  Constant5/1 -> MATLAB Function1/3(conductancemaxima1)
  Memory2/1 -> Product3/1, Discrete-Time Integrator1/2, Integrator2/2
  MATLAB Function1/2(conductancemaximum) -> single exp EPSCs generator (recurrent synapse)/3(conductance maximum)
  Constant6/1 -> Integrator2/1
  Constant4/1 -> MATLAB Function1/2(decaytimes1)
  Constant7/1 -> MATLAB Function2/2(decaytimes2)
  Constant8/1 -> MATLAB Function2/3(conductancemaxima2)
  Floor2/1 -> Product3/2
  Integrator2/1 -> single exp IPSCs generator (ihibitory synapse)/1(event time)
  Discrete-Time Integrator1/1 -> MATLAB Function2/1(eventnoumber)

== system pattern_separation/stimulation (pattern generator) ==
  Constant : Constant  Value=inputset  SampleTime=-1
  Constant1 : Constant  SampleTime=-1
  Discrete-Time Integrator : DiscreteIntegrator  InitialCondition=1  SampleTime=-1  LimitOutput=on  UpperSaturationLimit=simulationtime  ICPrevOutput=DiscIntNeverNeededParam  ICPrevScaledInput=DiscIntNeverNeededParam
  MATLAB Function : MATLAB Function  TreatAsAtomicUnit=on
  To Workspace3 : ToWorkspace  VariableName=stim_rasterplot  SampleTime=-1
  iteration : Constant  Value=trace  SampleTime=-1
  stim : Outport
  wires:
  MATLAB Function/1(trigger) -> To Workspace3/1, stim/1
  Discrete-Time Integrator/1 -> MATLAB Function/2(integrator)
  Constant/1 -> MATLAB Function/3(spiketrains)
  Constant1/1 -> Discrete-Time Integrator/1
  iteration/1 -> MATLAB Function/1(iteration)

== system pattern_separation/PV+ interneuron 1/interneuron ==
  postsynaptic current : Inport
  AHP or ADP : Constant  Value=c2  SampleTime=-1
  AP threshold potential : Constant  Value=vt2  SampleTime=-1
  Add : Sum  Inputs=+-
  Add2 : Sum  Inputs=+-
  Add3 : Sum  Inputs=+-
  Constant1 : Constant  Value=d2  SampleTime=-1
  Gain1 : Gain  Gain=b2
  Gain2 : Gain  Gain=k2
  Integrator : Integrator  ExternalReset=rising  InitialCondition=d2
  Integrator1 : Integrator  ExternalReset=rising  InitialCondition=vr2  LimitOutput=on  UpperSaturationLimit=30  LowerSaturationLimit=minimum_saturation_limit_2
  Memory : Memory  InheritSampleTime=on
  Memory1 : Memory  InitialCondition=vr2  InheritSampleTime=on
  Product : Product
  f' : Sum  Inputs=++-
  f'' : Sum  Inputs=+-
  membrne capacitance : Gain  Gain=1/C2(1)
  reset function : MATLAB Function  TreatAsAtomicUnit=on
  resting membrane potential : Constant  Value=vr2  SampleTime=-1
  time constant of relative refractory period : Gain  Gain=a2
  output : Outport
  wires:
  time constant of relative refractory period/1 -> Integrator/1  "u"
  Constant1/1 -> reset function/3(d)
  f''/1 -> time constant of relative refractory period/1
  membrne capacitance/1 -> Integrator1/1  "v"
  resting membrane potential/1 -> Add2/2, Add/2
  AHP or ADP/1 -> reset function/2(c)
  Add2/1 -> Product/1
  reset function/3(r) -> output/1, Integrator1/2, Integrator/2
  Gain1/1 -> f''/1
  Add3/1 -> Product/2
  Memory1/1 -> reset function/1(v)
  reset function/1(v1) -> Add/1, Add2/1, Add3/1
  reset function/2(u1) -> f''/2, f'/3
  Memory/1 -> reset function/4(u)
  Add/1 -> Gain1/1
  Integrator/1 -> Memory/1  "u"
  AP threshold potential/1 -> Add3/2
  Integrator1/1 -> Memory1/1  "v"
  f'/1 -> membrne capacitance/1
  Product/1 -> Gain2/1
  Gain2/1 -> f'/2
  postsynaptic current/1 -> f'/1

== system pattern_separation/PV+ interneuron 1/single exp EPSCs generator (ff synapse) ==
  event time : Inport
  decay time constant : Inport  Port=2
  conductance maximum : Inport  Port=3
  Add1 : Sum  Inputs=+-
  MATLAB Function : MATLAB Function  TreatAsAtomicUnit=on
  Multiply : Gain  Gain=-1
  Product : Product
  Product1 : Product  Inputs=*/
  Product2 : Product
  current reversal potential : Constant  Value=ve1  SampleTime=-1
  resting membrane potential : Constant  Value=vr1  SampleTime=-1
  postsynaptic current : Outport
  wires:
  decay time constant/1 -> Product1/2
  Product/1 -> postsynaptic current/1  "postsynaptic current"
  resting membrane potential/1 -> Add1/1
  current reversal potential/1 -> Add1/2
  conductance maximum/1 -> Product2/2
  Product2/1 -> Product/2  "conductance"
  Add1/1 -> Multiply/1
  Product1/1 -> MATLAB Function/1(inp)
  MATLAB Function/1(exponential) -> Product2/1
  event time/1 -> Product1/1
  Multiply/1 -> Product/1
